simulink model "hw2pendulum"  (R2013b)
settings: Solver=ode45  StartTime=0.0  StopTime=100  RelTol=1e-3
settings Model: Creator=czhang  LastModifiedBy=czhang

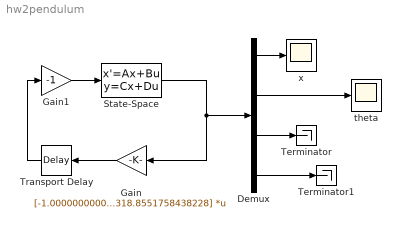
== system hw2pendulum ==
  Demux : Demux
  Gain : Gain  Gain="[-1.0000000000022 -325.6026451744055 -6.7416258738856  -318.8551758438228]"  Multiplication=Matrix(K*u)
  Gain1 : Gain  Gain=-1
  State-Space : StateSpace  A=[0 0 1 0; 0 0 0 1; 0 -9.8*1/10 0 0; 0 9.8*11/(10*10) 0 0]  B=[0; 0; 1/10; -1/(10*10)]  C=eye(4)  D=[0; 0; 0; 0]  X0=.5*[1 1 1 1]
  Terminator : Terminator
  Terminator1 : Terminator
  Transport Delay : TransportDelay  DelayTime=.4
  theta : Scope
  x : Scope
  wires:
  State-Space/1 -> Gain/1, Demux/1
  Demux/4 -> Terminator1/1
  Demux/3 -> Terminator/1
  Demux/2 -> theta/1
  Demux/1 -> x/1
  Gain/1 -> Transport Delay/1
  Transport Delay/1 -> Gain1/1
  Gain1/1 -> State-Space/1
